simulink model "MoonRoverNMSS"  (R2025b)
settings: Solver=ode15s  StartTime=0.0  StopTime=100000  RelTol=1e-3  AbsTol=1e-3
undefined symbols (not defined in the file): Area, Constant, Spec
libraries: fl_lib x50, nesl_utility x21, G_IR_function x7, G_solar_function x7
settings Model: DataDictionary=data_params.sldd  Creator=cdt  LastModifiedBy=cdt
settings SolverCC: AutoScaleAbsTol=off  AlgebraicLoopSolver=TrustRegion  MaxZcPerStep=1.0
settings DebuggingCC: UnconnectedInputMsg=warning  UnconnectedOutputMsg=warning  UnconnectedLineMsg=warning  SymbolicDimsDataTypeCodeGenerationDiagnostic=none
settings ModelReferenceCC: EnableRefExpFcnMdlSchedulingChecks=on
settings SFSimCC: CustomCodeUndefinedFunction=UseInterfaceOnly
settings RTWCC: GPUComputeCapability=3.5  DLArmComputeVersion=19.05
settings SimscapeCC: SimscapeLogType=all  SimscapeLogLimitData=off  SimscapeLogDataHistory=10000.0

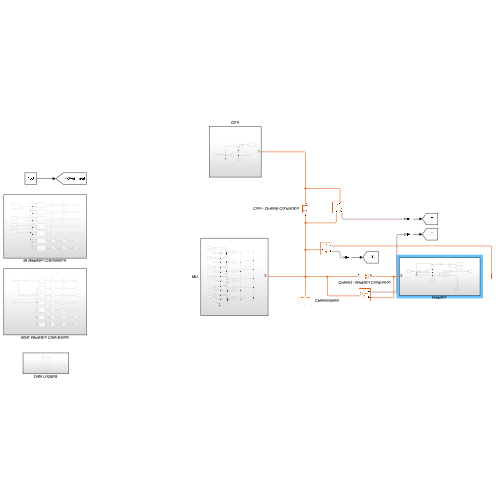
[thumbnail: Simulink's stored preview of the top-level diagram]
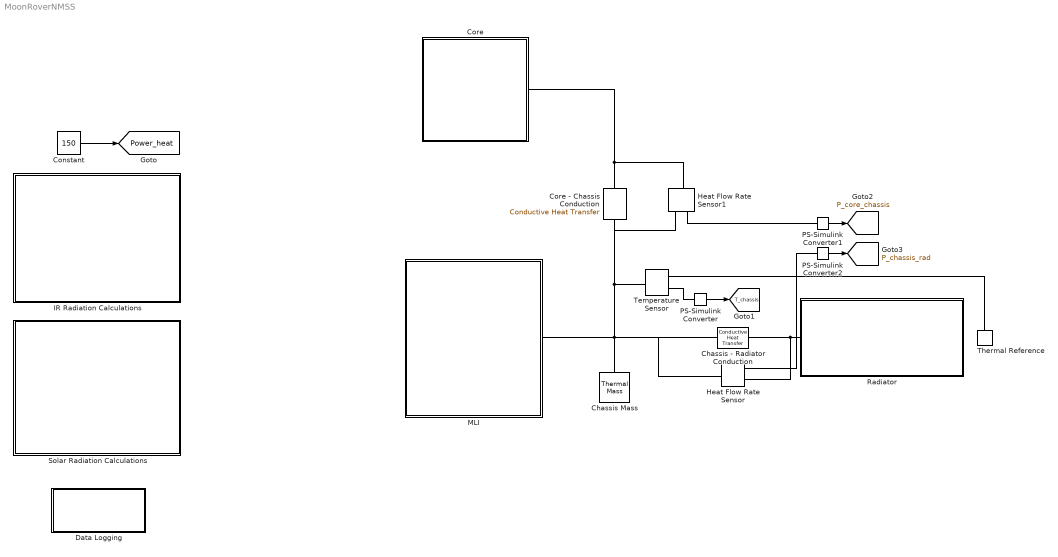
== system MoonRoverNMSS ==
  Chassis - Radiator Conduction : fl_lib/Thermal/Thermal Elements/Conductive Heat Transfer  thermal_type=foundation.enum.ConstantVariableTabulated.Constant  wall_geometry=foundation.enum.ConductionWallGeometry.Planar  area=Cond.area_chassis_rad m^2  thickness=Cond.thick_chassis_rad m  d_in=0.05 m  d_out=0.1 m  L=1 m  th_cond_min=10 W/(K*m)  th_cond=Cond.k_chassis_rad W/(K*m)  th_cond_TLU=[413, 401, 392, 383, 371, 357, 342] W/(K*m)  temp_TLU=[200, 273, 400, 600, 800, 1000, 1200] K  T_specify=off  T_priority=None  T=0 K  T_nominal_specify=off  T_nominal_value=1  T_nominal_unit=K  Q_specify=off  Q_priority=None  Q=0 W  Q_nominal_specify=off  Q_nominal_value=1  Q_nominal_unit=W
  Chassis Mass : fl_lib/Thermal/Thermal Elements/Thermal Mass  mass_type=foundation.enum.constant_variable.constant  mass=Spec.mass_chassis_kg kg  sp_heat=Spec.cp_chassis_J_kgK J/(K*kg)  mass_min=1e-6 kg  num_ports=foundation.enum.numPorts2.one  m_specify=off  m_priority=High  m=1 kg  m_nominal_specify=off  m_nominal_value=1  m_nominal_unit=kg  T_specify=on  T_priority=High  T=293 K  T_nominal_specify=off  T_nominal_value=1  T_nominal_unit=K  Q_specify=off  Q_priority=None  Q=0 W  Q_nominal_specify=off  Q_nominal_value=1  Q_nominal_unit=W
  Constant : Constant  Value=150
  Core : Subsystem
  Core - Chassis Conduction : fl_lib/Thermal/Thermal Elements/Conductive Heat Transfer  thermal_type=foundation.enum.ConstantVariableTabulated.Constant  wall_geometry=foundation.enum.ConductionWallGeometry.Planar  area=Cond.area_core_chassis m^2  thickness=Cond.thick_core_chassis m  d_in=0.05 m  d_out=0.1 m  L=1 m  th_cond_min=10 W/(K*m)  th_cond=Cond.k_core_chassis W/(K*m)  th_cond_TLU=[413, 401, 392, 383, 371, 357, 342] W/(K*m)  temp_TLU=[200, 273, 400, 600, 800, 1000, 1200] K  T_specify=off  T_priority=None  T=0 K  T_nominal_specify=off  T_nominal_value=1  T_nominal_unit=K  Q_specify=off  Q_priority=None  Q=0 W  Q_nominal_specify=off  Q_nominal_value=1  Q_nominal_unit=W
  Data Logging : Subsystem
  Heat Flow Rate Sensor : fl_lib/Thermal/Thermal Sensors/Heat Flow Rate Sensor
  Heat Flow Rate Sensor1 : fl_lib/Thermal/Thermal Sensors/Heat Flow Rate Sensor
  IR Radiation Calculations : Subsystem
  MLI : Subsystem
      settings: PortSchema="{\"entries\":[{\"content\":{\"sides\":[{\"content\":{},\"type\":\"ConnectorPlacement.EquallySpacedRectSide\",\"uuid\":\"d47134fd-2d2c-4c50-b6c5-63f88e3e0e34\"},{\"content\":{\"side\":\"RIGHT\"},\"type\":\"ConnectorPlacement.EquallySpacedRectSide\",\"uuid\":\"923c09c8-b9a5-46f2-be61-1fea53404d69\"},{\"content\":{\"connectorIds\":[\"LConn1\"],\"side\":\"TOP\"},\"type\":\"ConnectorPlacement.EquallySpacedRectSide\",\"uuid\":\"df6cd953-e26d-43a4-8b53-09965b1666ee\"}]},\"type\":\"ConnectorPlacement.EquallySpacedConnector\",\"uuid\":\"c91a916a-b2f4-4965-88a2-053ea405b0b3\"}],\"packageUris\":[\"http://schema.mathworks.com/mf0/Connector/R2020b\"],\"version\":\"1.0\"}"
  PS-Simulink Converter : nesl_utility/PS-Simulink Converter  PhysicalDomain=network_engine_domain  SubClassName=ps_output  LeftPortType=input  RightPortType=output  PseudoPeriodic=off  Frequencies=[]  VectorFormat=inherit  Unit=inherit  AffineConversion=off
  PS-Simulink Converter1 : nesl_utility/PS-Simulink Converter  PhysicalDomain=network_engine_domain  SubClassName=ps_output  LeftPortType=input  RightPortType=output  PseudoPeriodic=off  Frequencies=[]  VectorFormat=inherit  Unit=inherit  AffineConversion=off
  PS-Simulink Converter2 : nesl_utility/PS-Simulink Converter  PhysicalDomain=network_engine_domain  SubClassName=ps_output  LeftPortType=input  RightPortType=output  PseudoPeriodic=off  Frequencies=[]  VectorFormat=inherit  Unit=inherit  AffineConversion=off
  Radiator : Subsystem
  Solar Radiation Calculations : Subsystem
  Temperature Sensor : fl_lib/Thermal/Thermal Sensors/Temperature Sensor  temperature_measure=foundation.enum.MeasurementReference.difference
  Thermal Reference : fl_lib/Thermal/Thermal Elements/Thermal Reference
  tag scope: P_chassis_rad=global, P_core_chassis=global, Power_heat=global, T_chassis=global
  wires:
  Constant/1 -> [Power_heat]
  PS-Simulink Converter/1 -> [T_chassis]
  PS-Simulink Converter2/1 -> [P_chassis_rad]
  PS-Simulink Converter1/1 -> [P_core_chassis]
  connections:
  Chassis - Radiator Conduction/RConn1 -- Heat Flow Rate Sensor/RConn2 -- Radiator/LConn1
  Core/LConn1 -- Core - Chassis Conduction/LConn1 -- Heat Flow Rate Sensor1/LConn1
  MLI/LConn1 -- Heat Flow Rate Sensor/LConn1 -- Chassis - Radiator Conduction/LConn1 -- Heat Flow Rate Sensor1/RConn2 -- Core - Chassis Conduction/RConn1 -- Temperature Sensor/LConn1 -- Chassis Mass/LConn1
  Thermal Reference/LConn1 -- Temperature Sensor/RConn1
  PS-Simulink Converter/LConn1 -- Temperature Sensor/RConn2
  Heat Flow Rate Sensor1/RConn1 -- PS-Simulink Converter1/LConn1
  Heat Flow Rate Sensor/RConn1 -- PS-Simulink Converter2/LConn1

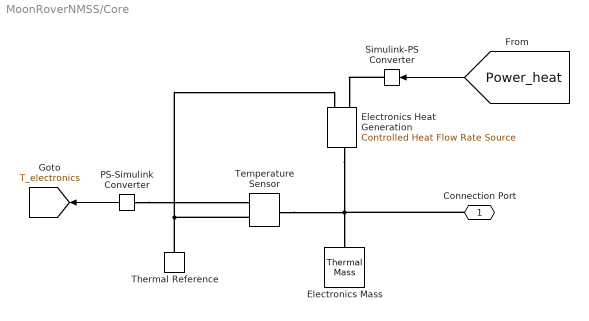
== system MoonRoverNMSS/Core ==
  Electronics Heat Generation : fl_lib/Thermal/Thermal Sources/Controlled Heat Flow Rate Source
  Electronics Mass : fl_lib/Thermal/Thermal Elements/Thermal Mass  mass_type=foundation.enum.constant_variable.constant  mass=Spec.mass_electronics_kg kg  sp_heat=Spec.cp_electronics_J_kgK J/(K*kg)  mass_min=1e-6 kg  num_ports=foundation.enum.numPorts2.one  m_specify=off  m_priority=High  m=1 kg  m_nominal_specify=off  m_nominal_value=1  m_nominal_unit=kg  T_specify=on  T_priority=High  T=293 K  T_nominal_specify=off  T_nominal_value=1  T_nominal_unit=K  Q_specify=off  Q_priority=None  Q=0 W  Q_nominal_specify=off  Q_nominal_value=1  Q_nominal_unit=W
  PS-Simulink Converter : nesl_utility/PS-Simulink Converter  PhysicalDomain=network_engine_domain  SubClassName=ps_output  LeftPortType=input  RightPortType=output  PseudoPeriodic=off  Frequencies=[]  VectorFormat=inherit  Unit=inherit  AffineConversion=off
  Simulink-PS Converter : nesl_utility/Simulink-PS Converter  PhysicalDomain=network_engine_domain  SubClassName=ps_input  LeftPortType=input  RightPortType=output  PseudoPeriodic=off  Frequencies=[]  NoiseDistribution=none  NoiseParameters=[]  Unit=1  AffineConversion=off  FilteringAndDerivatives=provide  SimscapeFilterOrder=1  InputFilterTimeConstant=0.001  UdotUserProvided=0
  Temperature Sensor : fl_lib/Thermal/Thermal Sensors/Temperature Sensor  temperature_measure=foundation.enum.MeasurementReference.difference
  Thermal Reference : fl_lib/Thermal/Thermal Elements/Thermal Reference
  Connection Port : PMIOPort  Side=Left
  tag scope: T_electronics=global
  wires:
  [Power_heat] -> Simulink-PS Converter/1
  PS-Simulink Converter/1 -> [T_electronics]
  connections:
  Connection Port/RConn1 -- Electronics Heat Generation/LConn1 -- Temperature Sensor/LConn1 -- Electronics Mass/LConn1
  Simulink-PS Converter/RConn1 -- Electronics Heat Generation/RConn1
  Thermal Reference/LConn1 -- Electronics Heat Generation/RConn2 -- Temperature Sensor/RConn1
  PS-Simulink Converter/LConn1 -- Temperature Sensor/RConn2

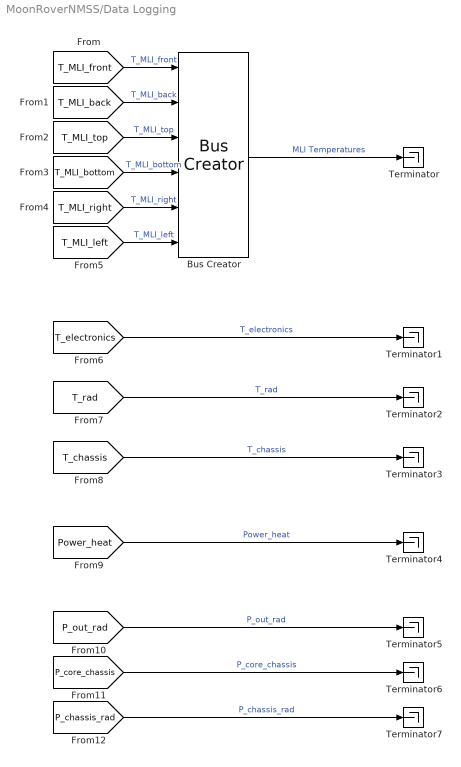
== system MoonRoverNMSS/Data Logging ==
  Bus Creator : BusCreator  Inputs=6
  Terminator{,1..7} (8 alike) : Terminator
  wires:
  [T_MLI_front] -> Bus Creator/1  "T_MLI_front"
  [T_MLI_back] -> Bus Creator/2  "T_MLI_back"
  [T_MLI_top] -> Bus Creator/3  "T_MLI_top"
  [T_MLI_bottom] -> Bus Creator/4  "T_MLI_bottom"
  [T_MLI_right] -> Bus Creator/5  "T_MLI_right"
  [T_MLI_left] -> Bus Creator/6  "T_MLI_left"
  Bus Creator/1 -> Terminator/1  "MLI Temperatures"
  [T_electronics] -> Terminator1/1  "T_electronics"
  [T_rad] -> Terminator2/1  "T_rad"
  [T_chassis] -> Terminator3/1  "T_chassis"
  [Power_heat] -> Terminator4/1  "Power_heat"
  [P_chassis_rad] -> Terminator7/1  "P_chassis_rad"
  [P_core_chassis] -> Terminator6/1  "P_core_chassis"
  [P_out_rad] -> Terminator5/1  "P_out_rad"

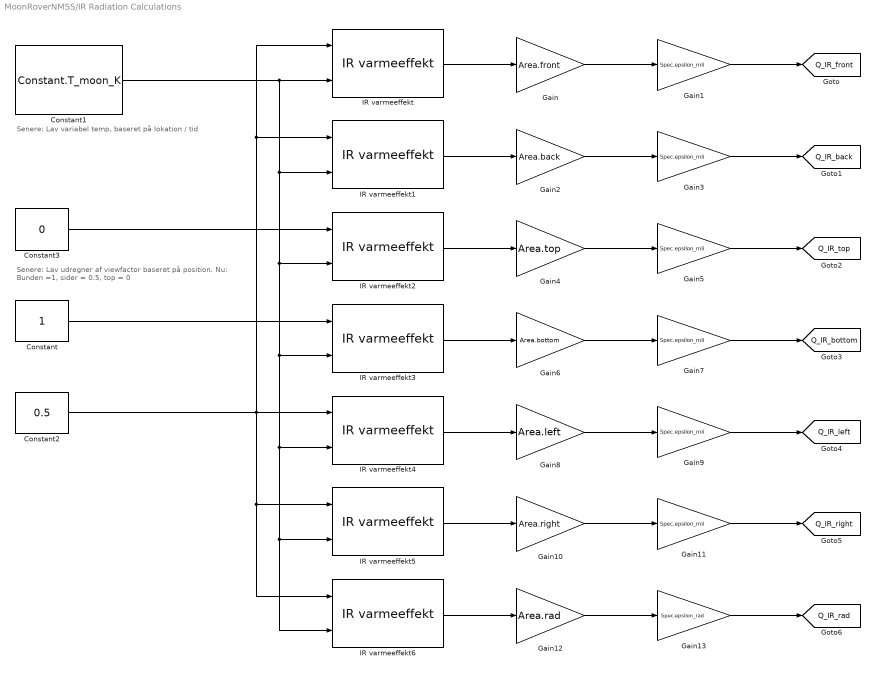
== system MoonRoverNMSS/IR Radiation Calculations ==
  note: Senere: Lav udregner af viewfactor baseret på position.
      | Nu: Bunden =1, sider = 0.5, top = 0
  note: Senere: Lav variabel temp, baseret på lokation / tid
   IR varmeeffekt{,1..6} (7 alike) : G_IR_function/ IR varmeeffekt  SystemSampleTime=-1  VariantActivationTime=update diagram  EmptyChoice=off  PassThrough=off  PassThroughVariantControl=(default)  EmptyChoiceVariantControl=(default)  AllowFlexibleInterface=on  Latency=0  AutoFrameSizeCalculation=off
  Constant : Constant
  Constant1 : Constant  Value=Constant.T_moon_K
  Constant2 : Constant  Value=0.5
  Constant3 : Constant  Value=0
  Gain : Gain  Gain=Area.front
  Gain{1,3,5,7,9,11} (6 alike) : Gain  Gain=Spec.epsilon_mli
  Gain10 : Gain  Gain=Area.right
  Gain12 : Gain  Gain=Area.rad
  Gain13 : Gain  Gain=Spec.epsilon_rad
  Gain2 : Gain  Gain=Area.back
  Gain4 : Gain  Gain=Area.top
  Gain6 : Gain  Gain=Area.bottom
  Gain8 : Gain  Gain=Area.left
  tag scope: Q_IR_back=global, Q_IR_bottom=global, Q_IR_front=global, Q_IR_left=global, Q_IR_rad=global, Q_IR_right=global, Q_IR_top=global
  wires:
  " IR varmeeffekt"/1 -> Gain/1
  Gain/1 -> Gain1/1
  Gain1/1 -> [Q_IR_front]
  Gain2/1 -> Gain3/1
  " IR varmeeffekt1"/1 -> Gain2/1
  Gain3/1 -> [Q_IR_back]
  Gain4/1 -> Gain5/1
  " IR varmeeffekt2"/1 -> Gain4/1
  Gain5/1 -> [Q_IR_top]
  Gain6/1 -> Gain7/1
  " IR varmeeffekt3"/1 -> Gain6/1
  Gain7/1 -> [Q_IR_bottom]
  Gain8/1 -> Gain9/1
  " IR varmeeffekt4"/1 -> Gain8/1
  Gain9/1 -> [Q_IR_left]
  Gain10/1 -> Gain11/1
  " IR varmeeffekt5"/1 -> Gain10/1
  Gain11/1 -> [Q_IR_right]
  Gain12/1 -> Gain13/1
  " IR varmeeffekt6"/1 -> Gain12/1
  Gain13/1 -> [Q_IR_rad]
  Constant1/1 -> " IR varmeeffekt1"/2, " IR varmeeffekt2"/2, " IR varmeeffekt3"/2, " IR varmeeffekt4"/2, " IR varmeeffekt5"/2, " IR varmeeffekt6"/2, " IR varmeeffekt"/2
  Constant/1 -> " IR varmeeffekt3"/1
  Constant3/1 -> " IR varmeeffekt2"/1
  Constant2/1 -> " IR varmeeffekt1"/1, " IR varmeeffekt"/1, " IR varmeeffekt5"/1, " IR varmeeffekt6"/1, " IR varmeeffekt4"/1

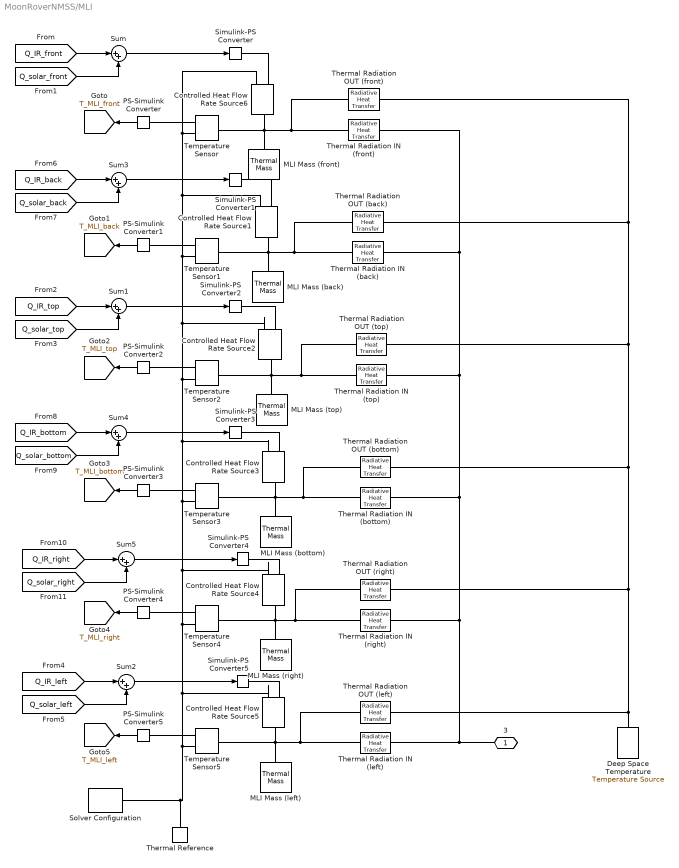
== system MoonRoverNMSS/MLI ==
  Controlled Heat Flow Rate Source{1..6} (6 alike) : fl_lib/Thermal/Thermal Sources/Controlled Heat Flow Rate Source
  Deep Space Temperature : fl_lib/Thermal/Thermal Sources/Temperature Source  temperature=3 K
  MLI Mass (back) : fl_lib/Thermal/Thermal Elements/Thermal Mass  mass_type=foundation.enum.constant_variable.constant  mass=Spec.mass_mli/6 kg  sp_heat=Spec.cp_mli_J_kgK J/(K*kg)  mass_min=1e-6 kg  num_ports=foundation.enum.numPorts2.one  m_specify=off  m_priority=High  m=1 kg  m_nominal_specify=off  m_nominal_value=1  m_nominal_unit=kg  T_specify=on  T_priority=High  T=220 K  T_nominal_specify=off  T_nominal_value=1  T_nominal_unit=K  Q_specify=off  Q_priority=None  Q=0 W  Q_nominal_specify=off  Q_nominal_value=1  Q_nominal_unit=W
  MLI Mass (bottom) : fl_lib/Thermal/Thermal Elements/Thermal Mass  mass_type=foundation.enum.constant_variable.constant  mass=Spec.mass_mli/6 kg  sp_heat=Spec.cp_mli_J_kgK J/(K*kg)  mass_min=1e-6 kg  num_ports=foundation.enum.numPorts2.one  m_specify=off  m_priority=High  m=1 kg  m_nominal_specify=off  m_nominal_value=1  m_nominal_unit=kg  T_specify=on  T_priority=High  T=220 K  T_nominal_specify=off  T_nominal_value=1  T_nominal_unit=K  Q_specify=off  Q_priority=None  Q=0 W  Q_nominal_specify=off  Q_nominal_value=1  Q_nominal_unit=W
  MLI Mass (front) : fl_lib/Thermal/Thermal Elements/Thermal Mass  mass_type=foundation.enum.constant_variable.constant  mass=Spec.mass_mli/6 kg  sp_heat=Spec.cp_mli_J_kgK J/(K*kg)  mass_min=1e-6 kg  num_ports=foundation.enum.numPorts2.one  m_specify=off  m_priority=High  m=1 kg  m_nominal_specify=off  m_nominal_value=1  m_nominal_unit=kg  T_specify=on  T_priority=High  T=220 K  T_nominal_specify=off  T_nominal_value=1  T_nominal_unit=K  Q_specify=off  Q_priority=None  Q=0 W  Q_nominal_specify=off  Q_nominal_value=1  Q_nominal_unit=W
  MLI Mass (left) : fl_lib/Thermal/Thermal Elements/Thermal Mass  mass_type=foundation.enum.constant_variable.constant  mass=Spec.mass_mli/6 kg  sp_heat=Spec.cp_mli_J_kgK J/(K*kg)  mass_min=1e-6 kg  num_ports=foundation.enum.numPorts2.one  m_specify=off  m_priority=High  m=1 kg  m_nominal_specify=off  m_nominal_value=1  m_nominal_unit=kg  T_specify=on  T_priority=High  T=220 K  T_nominal_specify=off  T_nominal_value=1  T_nominal_unit=K  Q_specify=off  Q_priority=None  Q=0 W  Q_nominal_specify=off  Q_nominal_value=1  Q_nominal_unit=W
  MLI Mass (right) : fl_lib/Thermal/Thermal Elements/Thermal Mass  mass_type=foundation.enum.constant_variable.constant  mass=Spec.mass_mli/6 kg  sp_heat=Spec.cp_mli_J_kgK J/(K*kg)  mass_min=1e-6 kg  num_ports=foundation.enum.numPorts2.one  m_specify=off  m_priority=High  m=1 kg  m_nominal_specify=off  m_nominal_value=1  m_nominal_unit=kg  T_specify=on  T_priority=High  T=220 K  T_nominal_specify=off  T_nominal_value=1  T_nominal_unit=K  Q_specify=off  Q_priority=None  Q=0 W  Q_nominal_specify=off  Q_nominal_value=1  Q_nominal_unit=W
  MLI Mass (top) : fl_lib/Thermal/Thermal Elements/Thermal Mass  mass_type=foundation.enum.constant_variable.constant  mass=Spec.mass_mli/6 kg  sp_heat=Spec.cp_mli_J_kgK J/(K*kg)  mass_min=1e-6 kg  num_ports=foundation.enum.numPorts2.one  m_specify=off  m_priority=High  m=1 kg  m_nominal_specify=off  m_nominal_value=1  m_nominal_unit=kg  T_specify=on  T_priority=High  T=220 K  T_nominal_specify=off  T_nominal_value=1  T_nominal_unit=K  Q_specify=off  Q_priority=None  Q=0 W  Q_nominal_specify=off  Q_nominal_value=1  Q_nominal_unit=W
  PS-Simulink Converter{,1..5} (6 alike) : nesl_utility/PS-Simulink Converter  PhysicalDomain=network_engine_domain  SubClassName=ps_output  LeftPortType=input  RightPortType=output  PseudoPeriodic=off  Frequencies=[]  VectorFormat=inherit  Unit=inherit  AffineConversion=off
  Simulink-PS Converter{,1..5} (6 alike) : nesl_utility/Simulink-PS Converter  PhysicalDomain=network_engine_domain  SubClassName=ps_input  LeftPortType=input  RightPortType=output  PseudoPeriodic=off  Frequencies=[]  NoiseDistribution=none  NoiseParameters=[]  Unit=1  AffineConversion=off  FilteringAndDerivatives=provide  SimscapeFilterOrder=1  InputFilterTimeConstant=0.001  UdotUserProvided=0
  Solver Configuration : nesl_utility/Solver Configuration  PhysicalDomain=network_engine_domain  SubClassName=solver  LeftPortType=input  RightPortType=generic  Tones=[]  Harmonics=[]  SimulateNoise=off  Profile=off  UseLocalSampling=off  EnableSwitchedLinearOptims=on  FrequencyDomain=off  UseCCode=off  RelTol=0.001  AbsTol=0.001  MinStep=1e-09  ToWorkspace=off  RevertToSquareIcSolve=off  NumHomotopyIterations=100  PhasorMode=off  PhasorModeNumHarmonics=1  ConsistencySolver=NEWTON_XTOL_AFTER_FTOL  IndexReductionMethod=DerivativeReplacement  DoDC=off  ResidualTolerance=1e-09  ConsistencyTolSource=GLOBAL  ConsistencyAbsTol=0.001  ConsistencyRelTol=0.001  ConsistencyTolFactor=0.001  UseLocalSolver=off  LocalSolverChoice=NE_BACKWARD_EULER_ADVANCER  ResolveIndetEquations=on  FunctionEvalNumThread=1  LocalSolverSampleTime=0.001  DoFixedCost=off  MaxNonlinIter=3  MaxModeIter=2  ComputeImpulses=off  ImpulseIterations=2  LinearAlgebra=auto  LinearAlgebraNumThread=0  EquationFormulation=NE_TIME_EF  DelaysMemoryBudget=1024  AutomaticFiltering=on  FilteringTimeConstant=0.001  PartitionStorageMethod=AS_NEEDED  PartitionMemoryBudget=1024  PartitionMethod=ROBUST  MultibodyUseLocalSolver=off  MultibodyLocalSolverChoice=ODE1  MultibodyLocalSolverSampleTime=0.001
  Sum{,1..5} (6 alike) : Sum  Inputs=|++
  Temperature Sensor{,1..5} (6 alike) : fl_lib/Thermal/Thermal Sensors/Temperature Sensor  temperature_measure=foundation.enum.MeasurementReference.difference
  Thermal Radiation IN (back) : fl_lib/Thermal/Thermal Elements/Radiative Heat Transfer  area=Area.back m^2  rad_tr_coeff=Constant.sigma * Spec.epsilon_eff_leak_mli W/(K^4*m^2)  T_specify=off  T_priority=None  T=0 K  T_nominal_specify=off  T_nominal_value=1  T_nominal_unit=K  Q_specify=off  Q_priority=None  Q=0 W  Q_nominal_specify=off  Q_nominal_value=1  Q_nominal_unit=W
      settings: InternalSimscapePortConfiguration="{\"Bottom\":[],\"Left\":[{\"id\":\"A\",\"label\":\"A\",\"type\":\"foundation.thermal.thermal\"}],\"Right\":[{\"id\":\"B\",\"label\":\"B\",\"type\":\"foundation.thermal.thermal\"}],\"Top\":[]}"
  Thermal Radiation IN (bottom) : fl_lib/Thermal/Thermal Elements/Radiative Heat Transfer  area=Area.bottom m^2  rad_tr_coeff=Constant.sigma * Spec.epsilon_eff_leak_mli W/(K^4*m^2)  T_specify=off  T_priority=None  T=0 K  T_nominal_specify=off  T_nominal_value=1  T_nominal_unit=K  Q_specify=off  Q_priority=None  Q=0 W  Q_nominal_specify=off  Q_nominal_value=1  Q_nominal_unit=W
      settings: InternalSimscapePortConfiguration="{\"Bottom\":[],\"Left\":[{\"id\":\"A\",\"label\":\"A\",\"type\":\"foundation.thermal.thermal\"}],\"Right\":[{\"id\":\"B\",\"label\":\"B\",\"type\":\"foundation.thermal.thermal\"}],\"Top\":[]}"
  Thermal Radiation IN (front) : fl_lib/Thermal/Thermal Elements/Radiative Heat Transfer  area=Area.front m^2  rad_tr_coeff=Constant.sigma * Spec.epsilon_eff_leak_mli W/(K^4*m^2)  T_specify=off  T_priority=None  T=0 K  T_nominal_specify=off  T_nominal_value=1  T_nominal_unit=K  Q_specify=off  Q_priority=None  Q=0 W  Q_nominal_specify=off  Q_nominal_value=1  Q_nominal_unit=W
      settings: InternalSimscapePortConfiguration="{\"Bottom\":[],\"Left\":[{\"id\":\"A\",\"label\":\"A\",\"type\":\"foundation.thermal.thermal\"}],\"Right\":[{\"id\":\"B\",\"label\":\"B\",\"type\":\"foundation.thermal.thermal\"}],\"Top\":[]}"
  Thermal Radiation IN (left) : fl_lib/Thermal/Thermal Elements/Radiative Heat Transfer  area=Area.left m^2  rad_tr_coeff=Constant.sigma * Spec.epsilon_eff_leak_mli W/(K^4*m^2)  T_specify=off  T_priority=None  T=0 K  T_nominal_specify=off  T_nominal_value=1  T_nominal_unit=K  Q_specify=off  Q_priority=None  Q=0 W  Q_nominal_specify=off  Q_nominal_value=1  Q_nominal_unit=W
      settings: InternalSimscapePortConfiguration="{\"Bottom\":[],\"Left\":[{\"id\":\"A\",\"label\":\"A\",\"type\":\"foundation.thermal.thermal\"}],\"Right\":[{\"id\":\"B\",\"label\":\"B\",\"type\":\"foundation.thermal.thermal\"}],\"Top\":[]}"
  Thermal Radiation IN (right) : fl_lib/Thermal/Thermal Elements/Radiative Heat Transfer  area=Area.right m^2  rad_tr_coeff=Constant.sigma * Spec.epsilon_eff_leak_mli W/(K^4*m^2)  T_specify=off  T_priority=None  T=0 K  T_nominal_specify=off  T_nominal_value=1  T_nominal_unit=K  Q_specify=off  Q_priority=None  Q=0 W  Q_nominal_specify=off  Q_nominal_value=1  Q_nominal_unit=W
      settings: InternalSimscapePortConfiguration="{\"Bottom\":[],\"Left\":[{\"id\":\"A\",\"label\":\"A\",\"type\":\"foundation.thermal.thermal\"}],\"Right\":[{\"id\":\"B\",\"label\":\"B\",\"type\":\"foundation.thermal.thermal\"}],\"Top\":[]}"
  Thermal Radiation IN (top) : fl_lib/Thermal/Thermal Elements/Radiative Heat Transfer  area=Area.top m^2  rad_tr_coeff=Constant.sigma * Spec.epsilon_eff_leak_mli W/(K^4*m^2)  T_specify=off  T_priority=None  T=0 K  T_nominal_specify=off  T_nominal_value=1  T_nominal_unit=K  Q_specify=off  Q_priority=None  Q=0 W  Q_nominal_specify=off  Q_nominal_value=1  Q_nominal_unit=W
      settings: InternalSimscapePortConfiguration="{\"Bottom\":[],\"Left\":[{\"id\":\"A\",\"label\":\"A\",\"type\":\"foundation.thermal.thermal\"}],\"Right\":[{\"id\":\"B\",\"label\":\"B\",\"type\":\"foundation.thermal.thermal\"}],\"Top\":[]}"
  Thermal Radiation OUT (back) : fl_lib/Thermal/Thermal Elements/Radiative Heat Transfer  area=Area.back m^2  rad_tr_coeff=Constant.sigma * Spec.epsilon_mli W/(K^4*m^2)  T_specify=off  T_priority=None  T=0 K  T_nominal_specify=off  T_nominal_value=1  T_nominal_unit=K  Q_specify=off  Q_priority=None  Q=0 W  Q_nominal_specify=off  Q_nominal_value=1  Q_nominal_unit=W
      settings: InternalSimscapePortConfiguration="{\"Bottom\":[],\"Left\":[{\"id\":\"A\",\"label\":\"A\",\"type\":\"foundation.thermal.thermal\"}],\"Right\":[{\"id\":\"B\",\"label\":\"B\",\"type\":\"foundation.thermal.thermal\"}],\"Top\":[]}"
  Thermal Radiation OUT (bottom) : fl_lib/Thermal/Thermal Elements/Radiative Heat Transfer  area=Area.bottom m^2  rad_tr_coeff=Constant.sigma * Spec.epsilon_mli W/(K^4*m^2)  T_specify=off  T_priority=None  T=0 K  T_nominal_specify=off  T_nominal_value=1  T_nominal_unit=K  Q_specify=off  Q_priority=None  Q=0 W  Q_nominal_specify=off  Q_nominal_value=1  Q_nominal_unit=W
      settings: InternalSimscapePortConfiguration="{\"Bottom\":[],\"Left\":[{\"id\":\"A\",\"label\":\"A\",\"type\":\"foundation.thermal.thermal\"}],\"Right\":[{\"id\":\"B\",\"label\":\"B\",\"type\":\"foundation.thermal.thermal\"}],\"Top\":[]}"
  Thermal Radiation OUT (front) : fl_lib/Thermal/Thermal Elements/Radiative Heat Transfer  area=Area.front m^2  rad_tr_coeff=Constant.sigma * Spec.epsilon_mli W/(K^4*m^2)  T_specify=off  T_priority=None  T=0 K  T_nominal_specify=off  T_nominal_value=1  T_nominal_unit=K  Q_specify=off  Q_priority=None  Q=0 W  Q_nominal_specify=off  Q_nominal_value=1  Q_nominal_unit=W
      settings: InternalSimscapePortConfiguration="{\"Bottom\":[],\"Left\":[{\"id\":\"A\",\"label\":\"A\",\"type\":\"foundation.thermal.thermal\"}],\"Right\":[{\"id\":\"B\",\"label\":\"B\",\"type\":\"foundation.thermal.thermal\"}],\"Top\":[]}"
  Thermal Radiation OUT (left) : fl_lib/Thermal/Thermal Elements/Radiative Heat Transfer  area=Area.left m^2  rad_tr_coeff=Constant.sigma * Spec.epsilon_mli W/(K^4*m^2)  T_specify=off  T_priority=None  T=0 K  T_nominal_specify=off  T_nominal_value=1  T_nominal_unit=K  Q_specify=off  Q_priority=None  Q=0 W  Q_nominal_specify=off  Q_nominal_value=1  Q_nominal_unit=W
      settings: InternalSimscapePortConfiguration="{\"Bottom\":[],\"Left\":[{\"id\":\"A\",\"label\":\"A\",\"type\":\"foundation.thermal.thermal\"}],\"Right\":[{\"id\":\"B\",\"label\":\"B\",\"type\":\"foundation.thermal.thermal\"}],\"Top\":[]}"
  Thermal Radiation OUT (right) : fl_lib/Thermal/Thermal Elements/Radiative Heat Transfer  area=Area.right m^2  rad_tr_coeff=Constant.sigma * Spec.epsilon_mli W/(K^4*m^2)  T_specify=off  T_priority=None  T=0 K  T_nominal_specify=off  T_nominal_value=1  T_nominal_unit=K  Q_specify=off  Q_priority=None  Q=0 W  Q_nominal_specify=off  Q_nominal_value=1  Q_nominal_unit=W
      settings: InternalSimscapePortConfiguration="{\"Bottom\":[],\"Left\":[{\"id\":\"A\",\"label\":\"A\",\"type\":\"foundation.thermal.thermal\"}],\"Right\":[{\"id\":\"B\",\"label\":\"B\",\"type\":\"foundation.thermal.thermal\"}],\"Top\":[]}"
  Thermal Radiation OUT (top) : fl_lib/Thermal/Thermal Elements/Radiative Heat Transfer  area=Area.top m^2  rad_tr_coeff=Constant.sigma * Spec.epsilon_mli W/(K^4*m^2)  T_specify=off  T_priority=None  T=0 K  T_nominal_specify=off  T_nominal_value=1  T_nominal_unit=K  Q_specify=off  Q_priority=None  Q=0 W  Q_nominal_specify=off  Q_nominal_value=1  Q_nominal_unit=W
      settings: InternalSimscapePortConfiguration="{\"Bottom\":[],\"Left\":[{\"id\":\"A\",\"label\":\"A\",\"type\":\"foundation.thermal.thermal\"}],\"Right\":[{\"id\":\"B\",\"label\":\"B\",\"type\":\"foundation.thermal.thermal\"}],\"Top\":[]}"
  Thermal Reference : fl_lib/Thermal/Thermal Elements/Thermal Reference
  3 : PMIOPort  Side=Left
  tag scope: T_MLI_back=global, T_MLI_bottom=global, T_MLI_front=global, T_MLI_left=global, T_MLI_right=global, T_MLI_top=global
  wires:
  [Q_IR_front] -> Sum/1
  [Q_solar_front] -> Sum/2
  [Q_IR_top] -> Sum1/1
  [Q_solar_top] -> Sum1/2
  [Q_IR_left] -> Sum2/1
  [Q_solar_left] -> Sum2/2
  [Q_IR_back] -> Sum3/1
  [Q_solar_back] -> Sum3/2
  [Q_IR_bottom] -> Sum4/1
  [Q_solar_bottom] -> Sum4/2
  [Q_IR_right] -> Sum5/1
  [Q_solar_right] -> Sum5/2
  Sum/1 -> Simulink-PS Converter/1
  Sum1/1 -> Simulink-PS Converter2/1
  Sum2/1 -> Simulink-PS Converter5/1
  Sum3/1 -> Simulink-PS Converter1/1
  Sum4/1 -> Simulink-PS Converter3/1
  Sum5/1 -> Simulink-PS Converter4/1
  PS-Simulink Converter/1 -> [T_MLI_front]
  PS-Simulink Converter1/1 -> [T_MLI_back]
  PS-Simulink Converter2/1 -> [T_MLI_top]
  PS-Simulink Converter3/1 -> [T_MLI_bottom]
  PS-Simulink Converter4/1 -> [T_MLI_right]
  PS-Simulink Converter5/1 -> [T_MLI_left]
  connections:
  Simulink-PS Converter/RConn1 -- Controlled Heat Flow Rate Source6/RConn1
  Simulink-PS Converter1/RConn1 -- Controlled Heat Flow Rate Source1/RConn1
  Simulink-PS Converter2/RConn1 -- Controlled Heat Flow Rate Source2/RConn1
  Simulink-PS Converter3/RConn1 -- Controlled Heat Flow Rate Source3/RConn1
  Simulink-PS Converter4/RConn1 -- Controlled Heat Flow Rate Source4/RConn1
  Simulink-PS Converter5/RConn1 -- Controlled Heat Flow Rate Source5/RConn1
  Solver Configuration/RConn1 -- Temperature Sensor1/RConn1 -- Temperature Sensor/RConn1 -- Controlled Heat Flow Rate Source6/RConn2 -- Controlled Heat Flow Rate Source1/RConn2 -- Controlled Heat Flow Rate Source2/RConn2 -- Temperature Sensor2/RConn1 -- Controlled Heat Flow Rate Source3/RConn2 -- Temperature Sensor3/RConn1 -- Controlled Heat Flow Rate Source4/RConn2 -- Temperature Sensor4/RConn1 -- Controlled Heat Flow Rate Source5/RConn2 -- Temperature Sensor5/RConn1 -- Thermal Reference/LConn1
  3/RConn1 -- Thermal Radiation IN (right)/RConn1 -- Thermal Radiation IN (bottom)/RConn1 -- Thermal Radiation IN (top)/RConn1 -- Thermal Radiation IN (front)/RConn1 -- Thermal Radiation IN (back)/RConn1 -- Thermal Radiation IN (left)/RConn1
  Controlled Heat Flow Rate Source5/LConn1 -- Temperature Sensor5/LConn1 -- Thermal Radiation OUT (left)/LConn1 -- Thermal Radiation IN (left)/LConn1 -- MLI Mass (left)/LConn1
  Controlled Heat Flow Rate Source4/LConn1 -- MLI Mass (right)/LConn1 -- Temperature Sensor4/LConn1 -- Thermal Radiation OUT (right)/LConn1 -- Thermal Radiation IN (right)/LConn1
  Controlled Heat Flow Rate Source3/LConn1 -- MLI Mass (bottom)/LConn1 -- Temperature Sensor3/LConn1 -- Thermal Radiation OUT (bottom)/LConn1 -- Thermal Radiation IN (bottom)/LConn1
  Controlled Heat Flow Rate Source2/LConn1 -- MLI Mass (top)/LConn1 -- Temperature Sensor2/LConn1 -- Thermal Radiation OUT (top)/LConn1 -- Thermal Radiation IN (top)/LConn1
  Controlled Heat Flow Rate Source1/LConn1 -- MLI Mass (back)/LConn1 -- Temperature Sensor1/LConn1 -- Thermal Radiation OUT (back)/LConn1 -- Thermal Radiation IN (back)/LConn1
  Thermal Radiation OUT (left)/RConn1 -- Thermal Radiation OUT (front)/RConn1 -- Thermal Radiation OUT (back)/RConn1 -- Thermal Radiation OUT (top)/RConn1 -- Thermal Radiation OUT (bottom)/RConn1 -- Thermal Radiation OUT (right)/RConn1 -- Deep Space Temperature/LConn1
  Thermal Radiation OUT (front)/LConn1 -- MLI Mass (front)/LConn1 -- Temperature Sensor/LConn1 -- Controlled Heat Flow Rate Source6/LConn1 -- Thermal Radiation IN (front)/LConn1
  Temperature Sensor/RConn2 -- PS-Simulink Converter/LConn1
  Temperature Sensor5/RConn2 -- PS-Simulink Converter5/LConn1
  Temperature Sensor4/RConn2 -- PS-Simulink Converter4/LConn1
  Temperature Sensor3/RConn2 -- PS-Simulink Converter3/LConn1
  Temperature Sensor2/RConn2 -- PS-Simulink Converter2/LConn1
  Temperature Sensor1/RConn2 -- PS-Simulink Converter1/LConn1

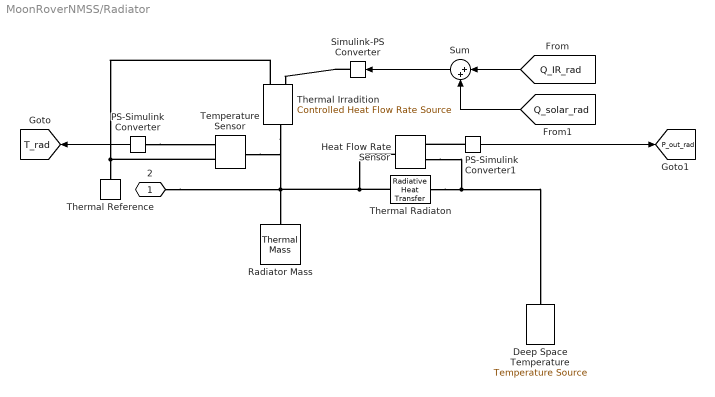
== system MoonRoverNMSS/Radiator ==
  Deep Space Temperature : fl_lib/Thermal/Thermal Sources/Temperature Source  temperature=3 K
  Heat Flow Rate Sensor : fl_lib/Thermal/Thermal Sensors/Heat Flow Rate Sensor
  PS-Simulink Converter : nesl_utility/PS-Simulink Converter  PhysicalDomain=network_engine_domain  SubClassName=ps_output  LeftPortType=input  RightPortType=output  PseudoPeriodic=off  Frequencies=[]  VectorFormat=inherit  Unit=inherit  AffineConversion=off
  PS-Simulink Converter1 : nesl_utility/PS-Simulink Converter  PhysicalDomain=network_engine_domain  SubClassName=ps_output  LeftPortType=input  RightPortType=output  PseudoPeriodic=off  Frequencies=[]  VectorFormat=inherit  Unit=inherit  AffineConversion=off
  Radiator Mass : fl_lib/Thermal/Thermal Elements/Thermal Mass  mass_type=foundation.enum.constant_variable.constant  mass=Spec.mass_rad_kg kg  sp_heat=Spec.cp_rad_J_kgK J/(K*kg)  mass_min=1e-6 kg  num_ports=foundation.enum.numPorts2.one  m_specify=off  m_priority=High  m=1 kg  m_nominal_specify=off  m_nominal_value=1  m_nominal_unit=kg  T_specify=on  T_priority=High  T=230 K  T_nominal_specify=off  T_nominal_value=1  T_nominal_unit=K  Q_specify=off  Q_priority=None  Q=0 W  Q_nominal_specify=off  Q_nominal_value=1  Q_nominal_unit=W
  Simulink-PS Converter : nesl_utility/Simulink-PS Converter  PhysicalDomain=network_engine_domain  SubClassName=ps_input  LeftPortType=input  RightPortType=output  PseudoPeriodic=off  Frequencies=[]  NoiseDistribution=none  NoiseParameters=[]  Unit=1  AffineConversion=off  FilteringAndDerivatives=provide  SimscapeFilterOrder=1  InputFilterTimeConstant=0.001  UdotUserProvided=0
  Sum : Sum  Inputs=|++
  Temperature Sensor : fl_lib/Thermal/Thermal Sensors/Temperature Sensor  temperature_measure=foundation.enum.MeasurementReference.difference
  Thermal Irradition : fl_lib/Thermal/Thermal Sources/Controlled Heat Flow Rate Source
  Thermal Radiaton : fl_lib/Thermal/Thermal Elements/Radiative Heat Transfer  area=Area.rad m^2  rad_tr_coeff=Constant.sigma * Spec.epsilon_rad W/(K^4*m^2)  T_specify=off  T_priority=None  T=0 K  T_nominal_specify=off  T_nominal_value=1  T_nominal_unit=K  Q_specify=off  Q_priority=None  Q=0 W  Q_nominal_specify=off  Q_nominal_value=1  Q_nominal_unit=W
      settings: InternalSimscapePortConfiguration="{\"Bottom\":[],\"Left\":[{\"id\":\"A\",\"label\":\"A\",\"type\":\"foundation.thermal.thermal\"}],\"Right\":[{\"id\":\"B\",\"label\":\"B\",\"type\":\"foundation.thermal.thermal\"}],\"Top\":[]}"
  Thermal Reference : fl_lib/Thermal/Thermal Elements/Thermal Reference
  2 : PMIOPort  Side=Left
  tag scope: P_out_rad=global, T_rad=global
  wires:
  Sum/1 -> Simulink-PS Converter/1
  [Q_solar_rad] -> Sum/2
  [Q_IR_rad] -> Sum/1
  PS-Simulink Converter/1 -> [T_rad]
  PS-Simulink Converter1/1 -> [P_out_rad]
  connections:
  Thermal Radiaton/RConn1 -- Heat Flow Rate Sensor/RConn2 -- Deep Space Temperature/LConn1
  Thermal Radiaton/LConn1 -- Heat Flow Rate Sensor/LConn1 -- Temperature Sensor/LConn1 -- Thermal Irradition/LConn1 -- 2/RConn1 -- Radiator Mass/LConn1
  Thermal Irradition/RConn2 -- Temperature Sensor/RConn1 -- Thermal Reference/LConn1
  Simulink-PS Converter/RConn1 -- Thermal Irradition/RConn1
  PS-Simulink Converter/LConn1 -- Temperature Sensor/RConn2
  PS-Simulink Converter1/LConn1 -- Heat Flow Rate Sensor/RConn1

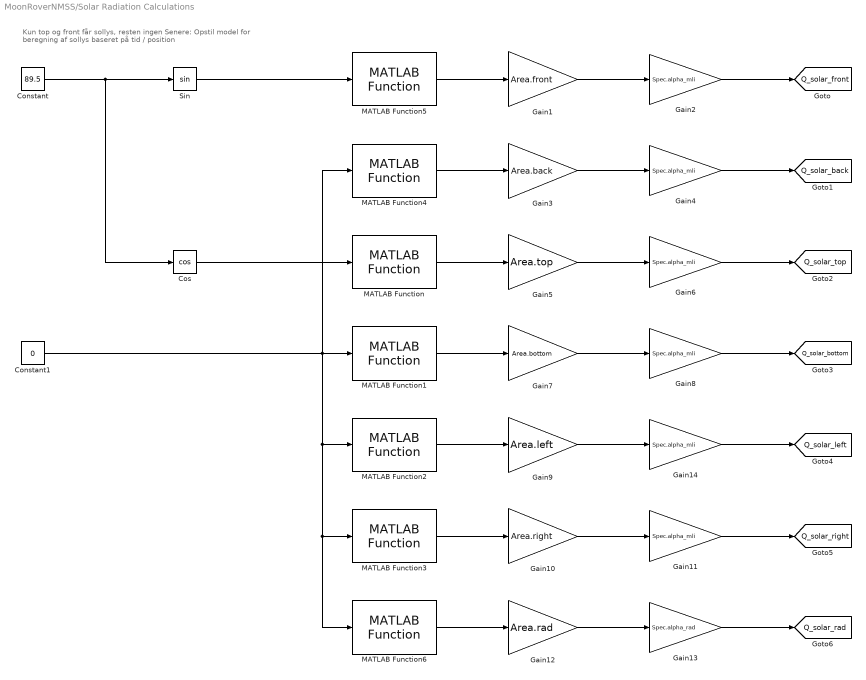
== system MoonRoverNMSS/Solar Radiation Calculations ==
  note: Kun top og front får sollys, resten ingen
      | Senere: Opstil model for beregning af sollys baseret på tid / position
  Constant : Constant  Value=89.5
  Constant1 : Constant  Value=0
  Cos : Trigonometry  Operator=cos
  Gain1 : Gain  Gain=Area.front
  Gain10 : Gain  Gain=Area.right
  Gain{2,4,6,8,11,14} (6 alike) : Gain  Gain=Spec.alpha_mli
  Gain12 : Gain  Gain=Area.rad
  Gain13 : Gain  Gain=Spec.alpha_rad
  Gain3 : Gain  Gain=Area.back
  Gain5 : Gain  Gain=Area.top
  Gain7 : Gain  Gain=Area.bottom
  Gain9 : Gain  Gain=Area.left
  MATLAB Function{,1..6} (7 alike) : G_solar_function/MATLAB Function  SystemSampleTime=-1  VariantActivationTime=update diagram  EmptyChoice=off  PassThrough=off  PassThroughVariantControl=(default)  EmptyChoiceVariantControl=(default)  AllowFlexibleInterface=on  Latency=0  AutoFrameSizeCalculation=off
  Sin : Trigonometry
  tag scope: Q_solar_back=global, Q_solar_bottom=global, Q_solar_front=global, Q_solar_left=global, Q_solar_rad=global, Q_solar_right=global, Q_solar_top=global
  wires:
  Gain10/1 -> Gain11/1
  MATLAB Function3/1 -> Gain10/1
  MATLAB Function4/1 -> Gain3/1
  Gain3/1 -> Gain4/1
  Gain6/1 -> [Q_solar_top]
  MATLAB Function/1 -> Gain5/1
  Gain5/1 -> Gain6/1
  Gain14/1 -> [Q_solar_left]
  Gain9/1 -> Gain14/1
  Gain4/1 -> [Q_solar_back]
  MATLAB Function2/1 -> Gain9/1
  MATLAB Function1/1 -> Gain7/1
  Gain7/1 -> Gain8/1
  MATLAB Function6/1 -> Gain12/1
  Gain13/1 -> [Q_solar_rad]
  Gain12/1 -> Gain13/1
  Gain11/1 -> [Q_solar_right]
  MATLAB Function5/1 -> Gain1/1
  Gain1/1 -> Gain2/1
  Gain2/1 -> [Q_solar_front]
  Gain8/1 -> [Q_solar_bottom]
  Constant/1 -> Sin/1, Cos/1
  Cos/1 -> MATLAB Function/1
  Sin/1 -> MATLAB Function5/1
  Constant1/1 -> MATLAB Function4/1, MATLAB Function2/1, MATLAB Function3/1, MATLAB Function6/1, MATLAB Function1/1
